simulink model "exp2_2019a"  (R2019a)
settings: Solver=ode4  StartTime=0.0  StopTime=20  FixedStep=0.001  MaxStep=0.01  RelTol=1e-3  AbsTol=1e-3  EnableMultiTasking=on
values from neighbouring files (symbols this model uses):
  a_1 = evalin('base','a_1')    [ik_pos2.m]
  a_2 = evalin('base','a_2')    [ik_pos2.m]
  a_3 = evalin('base','a_3')    [ik_pos2.m]
  b_0 = evalin('base','b_0')    [ik_pos2.m]    (also in ik_vel.m)
  b_1 = evalin('base','b_1')    [ik_pos2.m]
  b_2 = evalin('base','b_2')    [ik_pos2.m]
  I_1 = evalin('base','I_0')    [ik_vel.m]
  I_2 = evalin('base','I_0')    [ik_vel.m]
  I_3 = evalin('base','I_0')    [ik_vel.m]
  l_1 = evalin('base','l_1')    [ik_pos2.m]
  l_2 = evalin('base','l_2')    [ik_pos2.m]
  l_3 = evalin('base','l_3')    [ik_pos2.m]
  M = evalin('base','M')    [ik_pos2.m]
  m_0 = evalin('base','m_0')    [ik_pos2.m]
  m_1 = evalin('base','m_1')    [ik_pos2.m]
  m_2 = evalin('base','m_2')    [ik_pos2.m]
  m_3 = evalin('base','m_3')    [ik_pos2.m]
undefined symbols (not defined in the file or in its folder): b_3, I_0
settings Model: Creator=HP  LastModifiedBy=HP
settings SolverCC: AutoScaleAbsTol=off
settings DataIOCC: LimitDataPoints=on  MaxDataPoints=10000
settings OptimizationCC: LifeSpan=inf
settings DebuggingCC: AllowSymbolicDim=off  SFUnexpectedBacktrackingDiag=warning  SFNoUnconditionalDefaultTransitionDiag=warning  SFExecutionAtInitializationDiag=none  ArithmeticOperatorsInVariantConditions=warning
settings SFSimCC: SimUseLocalCustomCode=off
settings RTWCC: RTWUseLocalCustomCode=off
settings CodeAppCC: StateflowObjectComments=on
settings GRTTargetCC: TargetLangStandard=C89/C90 (ANSI)
settings ConfigComp: CovMetricSettings=dw  CovSaveCumulativeToWorkspaceVar=on  CovSaveSingleToWorkspaceVar=on  CovExternalEMLEnable=off  CovSFcnEnable=off
settings SimscapeCC: SimscapeLogType=all  SimscapeLogSimulationStatistics=on  SimscapeLogDataHistory=10000

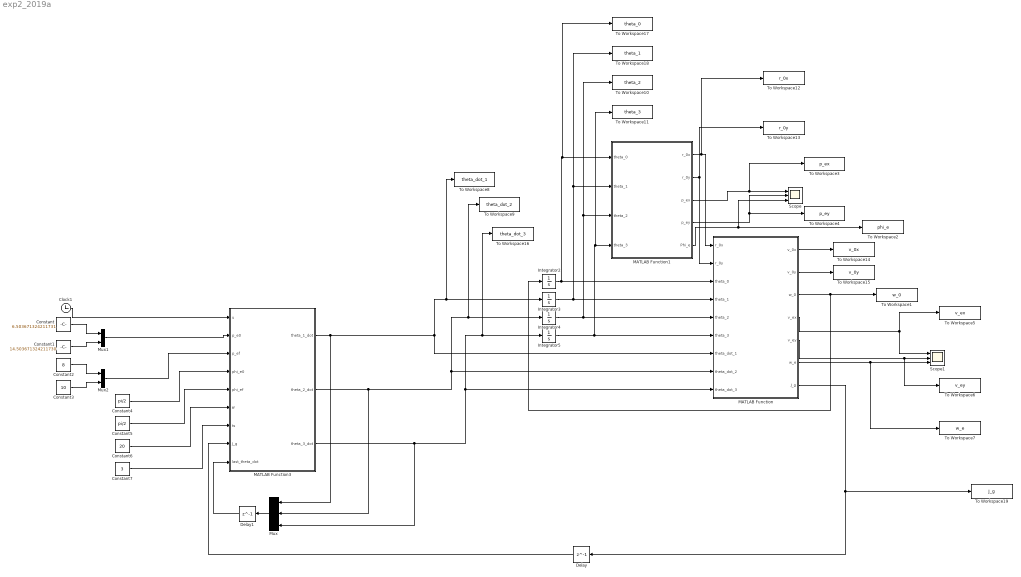
== system exp2_2019a ==
  Clock1 : Clock
  Constant : Constant  Value=6.503671324211731
  Constant1 : Constant  Value=14.503671324211730
  Constant2 : Constant  Value=8
  Constant3 : Constant  Value=10
  Constant4 : Constant  Value=pi/2
  Constant5 : Constant  Value=pi/2
  Constant6 : Constant  Value=20
  Constant7 : Constant  Value=3
  Delay : Delay  DelayLength=1  InitialCondition=0
  Delay1 : Delay  DelayLength=1  InitialCondition=0
  Integrator2 : Integrator
  Integrator3 : Integrator  InitialCondition=pi/4
  Integrator4 : Integrator  InitialCondition=pi/4
  Integrator5 : Integrator
  MATLAB Function : MATLAB Function  TreatAsAtomicUnit=on
  MATLAB Function1 : MATLAB Function  TreatAsAtomicUnit=on
  MATLAB Function3 : MATLAB Function  TreatAsAtomicUnit=on
  Mux : Mux  Inputs=3
  Mux1 : Mux  Inputs=2
  Mux2 : Mux  Inputs=2
  Scope : Scope  NumInputPorts=3
  Scope1 : Scope  NumInputPorts=3
  To Workspace1 : ToWorkspace  VariableName=w_0  SaveFormat=Timeseries  SampleTime=-1
  To Workspace10 : ToWorkspace  VariableName=theta_2  SaveFormat=Timeseries  SampleTime=-1
  To Workspace11 : ToWorkspace  VariableName=theta_3  SaveFormat=Timeseries  SampleTime=-1
  To Workspace12 : ToWorkspace  VariableName=r_0x  SaveFormat=Timeseries  SampleTime=-1
  To Workspace13 : ToWorkspace  VariableName=r_0y  SaveFormat=Timeseries  SampleTime=-1
  To Workspace14 : ToWorkspace  VariableName=v_0x  SaveFormat=Timeseries  SampleTime=-1
  To Workspace15 : ToWorkspace  VariableName=v_0y  SaveFormat=Timeseries  SampleTime=-1
  To Workspace16 : ToWorkspace  VariableName=theta_dot_3  SaveFormat=Timeseries  SampleTime=-1
  To Workspace17 : ToWorkspace  VariableName=theta_0  SaveFormat=Timeseries  SampleTime=-1
  To Workspace18 : ToWorkspace  VariableName=theta_1  SaveFormat=Timeseries  SampleTime=-1
  To Workspace19 : ToWorkspace  VariableName=J_g  SaveFormat=Timeseries  SampleTime=-1
  To Workspace2 : ToWorkspace  VariableName=phi_e  SaveFormat=Timeseries  SampleTime=-1
  To Workspace3 : ToWorkspace  VariableName=p_ex  SaveFormat=Timeseries  SampleTime=-1
  To Workspace4 : ToWorkspace  VariableName=p_ey  SaveFormat=Timeseries  SampleTime=-1
  To Workspace5 : ToWorkspace  VariableName=v_ex  SaveFormat=Timeseries  SampleTime=-1
  To Workspace6 : ToWorkspace  VariableName=v_ey  SaveFormat=Timeseries  SampleTime=-1
  To Workspace7 : ToWorkspace  VariableName=w_e  SaveFormat=Timeseries  SampleTime=-1
  To Workspace8 : ToWorkspace  VariableName=theta_dot_1  SaveFormat=Timeseries  SampleTime=-1
  To Workspace9 : ToWorkspace  VariableName=theta_dot_2  SaveFormat=Timeseries  SampleTime=-1
  wires:
  MATLAB Function/1(v_0x) -> To Workspace14/1
  MATLAB Function3/1(theta_1_dot) -> Mux/1, Integrator3/1, To Workspace8/1, MATLAB Function/7(theta_dot_1)
  MATLAB Function/2(v_0y) -> To Workspace15/1
  MATLAB Function3/2(theta_2_dot) -> Mux/2, To Workspace9/1, Integrator4/1, MATLAB Function/8(theta_dot_2)
  Integrator5/1 -> To Workspace11/1, MATLAB Function1/4(theta_3), MATLAB Function/6(theta_3)
  MATLAB Function/6(w_e) -> To Workspace7/1, Scope1/3
  MATLAB Function3/3(theta_3_dot) -> Mux/3, To Workspace16/1, Integrator5/1, MATLAB Function/9(theta_dot_3)
  MATLAB Function/5(v_ey) -> To Workspace6/1, Scope1/2
  MATLAB Function1/2(r_0y) -> MATLAB Function/2(r_0y), To Workspace13/1
  MATLAB Function1/1(r_0x) -> To Workspace12/1, MATLAB Function/1(r_0x)
  Integrator3/1 -> To Workspace18/1, MATLAB Function1/2(theta_1), MATLAB Function/4(theta_1)
  Integrator2/1 -> To Workspace17/1, MATLAB Function1/1(theta_0), MATLAB Function/3(theta_0)
  MATLAB Function/4(v_ex) -> Scope1/1, To Workspace5/1
  MATLAB Function1/4(p_ey) -> Scope/2, To Workspace4/1
  MATLAB Function1/3(p_ex) -> To Workspace3/1, Scope/1
  Integrator4/1 -> To Workspace10/1, MATLAB Function1/3(theta_2), MATLAB Function/5(theta_2)
  MATLAB Function1/5(Phi_e) -> Scope/3, To Workspace2/1
  Clock1/1 -> MATLAB Function3/1(u)
  Constant/1 -> Mux1/1
  Constant1/1 -> Mux1/2
  Mux1/1 -> MATLAB Function3/2(p_e0)
  Constant3/1 -> Mux2/2
  Mux2/1 -> MATLAB Function3/3(p_ef)
  Constant2/1 -> Mux2/1
  Constant4/1 -> MATLAB Function3/4(phi_e0)
  Constant5/1 -> MATLAB Function3/5(phi_ef)
  Constant6/1 -> MATLAB Function3/6(tf)
  Constant7/1 -> MATLAB Function3/7(ts)
  MATLAB Function/7(J_g) -> To Workspace19/1, Delay/1
  MATLAB Function/3(w_0) -> To Workspace1/1, Integrator2/1
  Delay/1 -> MATLAB Function3/8(J_g)
  Mux/1 -> Delay1/1
  Delay1/1 -> MATLAB Function3/9(last_theta_dot)

== matlab function exp2_2019a/MATLAB Function1 ==
  data: theta_0 input; r_0x output; theta_1 input; theta_2 input; theta_3 input; r_0y output; p_ex output; p_ey output; Phi_e output; a_1 parameter; a_2 parameter; a_3 parameter; b_0 parameter; b_1 parameter; b_2 parameter; b_3 parameter; l_1 parameter; l_2 parameter; l_3 parameter; m_0 parameter; m_1 parameter; m_2 parameter; m_3 parameter; M parameter; I_0 parameter; I_1 parameter; I_2 parameter; I_3 parameter
%根据公式6-294和6-295,6-296进行建模
function [r_0x,r_0y,p_ex,p_ey,Phi_e] = position(theta_0,theta_1,theta_2,theta_3, a_1, a_2, a_3, b_0, b_1, b_2, b_3, l_1, l_2, l_3, m_0, m_1, m_2, m_3, M, I_0, I_1, I_2, I_3)
    %读取工作空间的所有变量
%     a_1
%     a_1 = evalin('base','a_1');
%     a_2 = evalin('base','a_2');
%     a_3 = evalin('base','a_3');
%     b_0 = evalin('base','b_0');
%     b_1 = evalin('base','b_1');
%     b_2 = evalin('base','b_2');
%     b_3 = evalin('base','b_3');
%     l_1 = evalin('base','l_1');
%     l_2 = evalin('base','l_2');
%     l_3 = evalin('base','l_3');
%     m_0 = evalin('base','m_0');
%     m_1 = evalin('base','m_1');
%     m_2 = evalin('base','m_2');
%     m_3 = evalin('base','m_3');
%     M = evalin('base','M');
%     I_0 = evalin('base','I_0');
%     I_1 = evalin('base','I_0');
%     I_2 = evalin('base','I_0');
%     I_3 = evalin('base','I_0');
    
    %计算参数
    s_0 = sin(theta_0);
    c_0 = cos(theta_0);
    s_01 = sin(theta_0+theta_1);
    c_01 = cos(theta_0+theta_1);
    s_012 = sin(theta_0+theta_1+theta_2);
    c_012 = cos(theta_0+theta_1+theta_2);
    s_0123 = sin(theta_0+theta_1+theta_2+theta_3);
    c_0123 = cos(theta_0+theta_1+theta_2+theta_3);
    
    b_0_hat = m_0/M*b_0;
    b_1_hat = (m_0 + m_1)/M*b_1;
    b_2_hat = (m_0 + m_1 + m_2)/M*b_2;
    b_3_hat = b_2;

    a_1_hat = m_0/M*a_1;
    a_2_hat = (m_0+m_1)/M*a_2;
    a_3_hat = (m_0+m_1+m_2)/M*a_3;
    
    %计算r_0 公式6-293  check
    r_0x = -( (m_1+m_2+m_3)/M*b_0*c_0 + ((m_1+m_2+m_3)/M*a_1 + (m_2+m_3)/M*b_1)*c_01 + ((m_2+m_3)/M*a_2 + m_3/M*b_2)*c_012 + m_3/M*a_3*c_0123);
    r_0y = -( (m_1+m_2+m_3)/M*b_0*s_0 + ((m_1+m_2+m_3)/M*a_1 + (m_2+m_3)/M*b_1)*s_01 + ((m_2+m_3)/M*a_2 + m_3/M*b_2)*s_012 + m_3/M*a_3*s_0123);
    
    
    %计算末端位姿
    p_ex = b_0_hat*c_0 + (a_1_hat+b_1_hat)*c_01 + (a_2_hat+b_2_hat)*c_012+(a_3_hat+b_3_hat)*c_0123;
    p_ey = b_0_hat*s_0 + (a_1_hat+b_1_hat)*s_01 + (a_2_hat+b_2_hat)*s_012+(a_3_hat+b_3_hat)*s_0123;
    Phi_e = theta_0+theta_1+theta_2+theta_3;%末端姿态角

== matlab function exp2_2019a/MATLAB Function ==
  data: r_0x input; v_0x output; r_0y input; theta_0 input; theta_1 input; theta_2 input; theta_3 input; theta_dot_1 input; theta_dot_2 input; theta_dot_3 input; v_0y output; w_0 output; v_ex output; v_ey output; w_e output; a_1 parameter; a_2 parameter; a_3 parameter; b_0 parameter; b_1 parameter; b_2 parameter; b_3 parameter; l_1 parameter; l_2 parameter; l_3 parameter; m_0 parameter; m_1 parameter; m_2 parameter; m_3 parameter; M parameter; I_0 parameter; I_1 parameter; I_2 parameter; I_3 parameter; J_g output
%通过公式6-363计算末端速度
function [v_0x,v_0y,w_0,v_ex,v_ey,w_e,J_g] = velocity(r_0x,r_0y,theta_0,theta_1,theta_2,theta_3,theta_dot_1,theta_dot_2,theta_dot_3, a_1, a_2, a_3, b_0, b_1, b_2, b_3, l_1, l_2, l_3, m_0, m_1, m_2, m_3, M, I_0, I_1, I_2, I_3)
    %读取工作空间的所有变量
%     a_1 = evalin('base','a_1');
%     a_2 = evalin('base','a_2');
%     a_3 = evalin('base','a_3');
%     b_0 = evalin('base','b_0');
%     b_1 = evalin('base','b_1');
%     b_2 = evalin('base','b_2');
%     b_3 = evalin('base','b_3');
%     l_1 = evalin('base','l_1');
%     l_2 = evalin('base','l_2');
%     l_3 = evalin('base','l_3');
%     m_0 = evalin('base','m_0');
%     m_1 = evalin('base','m_1');
%     m_2 = evalin('base','m_2');
%     m_3 = evalin('base','m_3');
%     M = evalin('base','M');
%     I_0 = evalin('base','I_0');
%     I_1 = evalin('base','I_0');
%     I_2 = evalin('base','I_0');
%     I_3 = evalin('base','I_0');

    %更新各个参量
    s_0 = sin(theta_0);
    c_0 = cos(theta_0);
    s_01 = sin(theta_0+theta_1);
    c_01 = cos(theta_0+theta_1);
    s_012 = sin(theta_0+theta_1+theta_2);
    c_012 = cos(theta_0+theta_1+theta_2);
    s_0123 = sin(theta_0+theta_1+theta_2+theta_3);
    c_0123 = cos(theta_0+theta_1+theta_2+theta_3);

    k_vx = -m_1*(b_0*s_0+a_1*s_01)-m_2*(b_0*s_0+l_1*s_01+a_2*s_012)-m_3*(b_0*s_0+l_1*s_01+l_2*s_012+a_3*s_0123); %公式6-321    check
    k_vy = m_1*(b_0*c_0+a_1*c_01)+m_2*(b_0*c_0+l_1*c_01+a_2*c_012)+m_3*(b_0*c_0+l_1*c_01+l_2*c_012+a_3*c_0123); %公式6-322     check
    k_px1 = -m_1*a_1*s_01-m_2*(l_1*s_01+a_2*s_012)-m_3*(l_1*s_01+l_2*s_012+a_3*s_0123);%公式6-323   check
    k_px2 = -m_2*a_2*s_012 - m_3*(l_2*s_012+a_3*s_0123); %公式6-324   check
    k_px3 = -m_3*a_3*s_0123; %公式6-325    check

    k_py1 = m_1*a_1*c_01+m_2*(l_1*c_01+a_2*c_012)+m_3*(l_1*c_01+l_2*c_012+a_3*c_0123); %公式6-326   check
    k_py2 = m_2*a_2*c_012+m_3*(l_2*c_012+a_3*c_0123);  %公式6-327   check
    k_py3 = m_3*a_3*c_0123;  %公式6-328  check

    k_w = (I_0+I_1+I_2+I_3) + m_1*(b_0*c_0+a_1*c_01)^2 +m_1*(b_0*s_0+a_1*s_01)^2 ...
        +m_2*(b_0*c_0+l_1*c_01+a_2*c_012)^2+m_2*(b_0*s_0+l_1*s_01+a_2*s_012)^2 ...
        +m_2*(b_0*c_0+l_1*c_01+l_2*c_012+a_3*c_0123)^2 + m_3*(b_0*s_0+l_1*s_01+l_2*s_012+a_3*s_0123)^2 ...
        -M*(r_0x^2+r_0y^2); %公式6-353   check

    k_q1 = (I_1+I_2+I_3) +m_1*a_1*c_01*(b_0*c_0+a_1*c_01)+m_1*a_1*s_01*(b_0*s_0+a_1*s_01) ...
        +m_2*(l_1*c_01+a_2*c_012)*(b_0*c_0+l_1*c_01+a_2*c_012) ...
        +m_2*(l_1*s_01+a_2*s_012)*(b_0*s_0+l_1*s_01+a_2*s_012) ...
        +m_3*(l_1*c_01+l_2*c_012+a_3*c_0123)*(b_0*c_0+l_1*c_01+l_2*c_012+a_3*c_0123) ...
        +m_3*(l_1*s_01+l_2*s_012+a_3*s_0123)*(b_0*s_0+l_1*s_01+l_2*s_012+a_3*s_0123) ...
        +r_0x*(m_1*a_1*c_01+m_2*(l_1*c_01+a_2*c_012)+m_3*(l_1*c_01+l_2*c_012+a_3*c_0123)) ...
        +r_0y*(m_1*a_1*s_01+m_2*(l_1*s_01+a_2*s_012)+m_3*(l_1*s_01+l_2*s_012+a_3*s_0123)); %公式6-354    check

    k_q2 = (I_2+I_3)+m_2*a_2*c_012*(b_0*c_0+l_1*c_01+a_2*c_012)+m_2*a_2*s_012*(b_0*s_0+l_1*s_01+a_2*s_012) ...
        +m_3*(l_2*c_012+a_3*c_0123)*(b_0*c_0+l_1*c_01+l_2*c_012+a_3*c_0123) ...
        +m_3*(l_2*s_012+a_3*s_0123)*(b_0*s_0+l_1*s_01+l_2*s_012+a_3*s_0123) ...
        +r_0x*(m_2*a_2*c_012+m_3*(l_2*c_012+a_3*c_0123)) ...
        +r_0y*(m_2*a_2*s_012+m_3*(l_2*s_012+a_3*s_0123));%公式6-355     check

    k_q3 = I_3+m_3*a_3*c_0123*(b_0*c_0+l_1*c_01+l_2*c_012+a_3*c_0123)+m_3*a_3*s_0123*(b_0*s_0+l_1*s_01+l_2*s_012+a_3*s_0123) ...
        +m_3*a_3*c_0123*r_0x+m_3*a_3*s_0123*r_0y;%公式6-356     check

    J_s = [
        1     0     -b_0*s_0-l_1*s_01-l_2*s_012-l_3*s_0123;
        0     1      b_0*c_0+l_1*c_01+l_2*c_012+l_3*c_0123;
        0     0                        1                  ;
        ];%公式6-309   check
    J_m = [
        -l_1*s_01-l_2*s_012-l_3*s_0123  -l_2*s_012-l_3*s_0123    -l_3*s_0123;
         l_1*c_01+l_2*c_012+l_3*c_0123   l_2*c_012+l_3*c_0123     l_3*c_0123;
         1                               1                        1         ;
        ];  %公式6-310  check

    J_1 = [
        M   0   k_vx;
        0   M   k_vy;
        0   0   k_w ;
        ];%公式6-360  check
    J_2 = [
        k_px1  k_px2  k_px3;
        k_py1  k_py2  k_py3;
        k_q1   k_q2   k_q3
        ];%公式6-361   check
    J_g = -J_s*inv(J_1)*J_2+J_m;  %公式6-363  check

    
    %计算速度
    velocity_end = J_g*[theta_dot_1;theta_dot_2;theta_dot_3]; %末端速度
    velocity_0 = -inv(J_1)*J_2*[theta_dot_1;theta_dot_2;theta_dot_3];%基座速度
    v_ex = velocity_end(1);
    v_ey = velocity_end(2);
    w_e = velocity_end(3);
    v_0x = velocity_0(1);
    v_0y = velocity_0(2);
    w_0 = velocity_0(3);

== matlab function exp2_2019a/MATLAB Function3 ==
  data: u input; theta_1_dot output; p_e0 input; p_ef input; phi_e0 input; phi_ef input; tf input; ts input; J_g input; theta_2_dot output; theta_3_dot output; last_theta_dot input
function [theta_1_dot,theta_2_dot,theta_3_dot] = path_plan_continue(u,p_e0,p_ef,phi_e0,phi_ef, tf, ts, J_g,last_theta_dot)
%使用11.7.1章中的笛卡尔空间连续位姿跟踪的方法进行规划
    
    v_em = (p_ef-p_e0)/(tf-ts); %速度最大值
    
    w_em = (phi_ef-phi_e0)/(tf-ts); %角速度最大值
    
    %按照梯形函数输出
    
    if(u<ts)
        v_e = v_em/ts*u;
        w_e = w_em/ts*u;
    elseif(u < tf-ts)
        v_e = v_em;
        w_e = w_em;
        
    else
        v_e = v_em-v_em/ts*(u-tf+ts);
        w_e = w_em-w_em/ts*(u-tf+ts);
    end
    u
    v_ex = v_e(1)
    v_ey = v_e(2)
    w_e
    J_g
    %防止奇异

    if(det(J_g)==0)
        theta_1_dot = last_theta_dot(1);
        theta_2_dot = last_theta_dot(2);
        theta_3_dot = last_theta_dot(3);      
    else
        theta_dot = J_g\[v_ex,v_ey,w_e]';
        theta_1_dot = theta_dot(1);
        theta_2_dot = theta_dot(2);
        theta_3_dot = theta_dot(3);
    end
    




end
